simulink model "running_example"  (Simulink 10.0)
settings: Solver=ode45  StartTime=0.0  StopTime=50.0  RelTol=1e-3  EnableMultiTasking=on
settings Model: Creator=unknown  LastModifiedBy=bhisma
settings DataIOCC: LimitDataPoints=on  SignalLoggingSaveFormat=ModelDataLogs  SignalLoggingName=sigsOut
settings OptimizationCC: LifeSpan=auto
settings DebuggingCC: SaveWithParameterizedLinksMsg=none  SignalResolutionControl=TryResolveAllWithWarning  MultiTaskDSMMsg=warning  MultiTaskCondExecSysMsg=none  SFUnexpectedBacktrackingDiag=error  SFNoUnconditionalDefaultTransitionDiag=error  SFExecutionAtInitializationDiag=warning  ArithmeticOperatorsInVariantConditions=error
settings HardwareCC: TargetUnknown=on
settings SFSimCC: SimUseLocalCustomCode=on  CustomCodeUndefinedFunction=FilterOut
settings RTWCC: RTWUseLocalCustomCode=on
settings CodeAppCC: StateflowObjectComments=off
settings GRTTargetCC: TargetLangStandard=C99 (ISO)

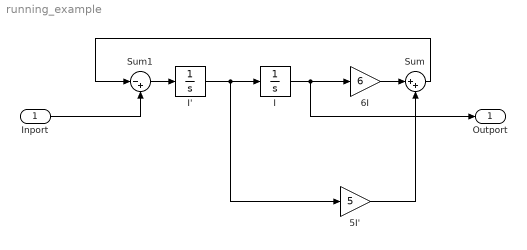
== system running_example ==
  Inport : Inport
  5I' : Gain  Gain=5  SaturateOnIntegerOverflow=on  OutDataTypeStr=Inherit: Same as input  ParamDataTypeStr=Inherit: Same as input
  6I : Gain  Gain=6  SaturateOnIntegerOverflow=on  OutDataTypeStr=Inherit: Same as input  ParamDataTypeStr=Inherit: Same as input
  I : Integrator  InitialCondition=1
  I' : Integrator  InitialCondition=5
  Sum : Sum  Inputs=|++  SaturateOnIntegerOverflow=on
  Sum1 : Sum  Inputs=|-+  SaturateOnIntegerOverflow=on
  Outport : Outport
  wires:
  I'/1 -> I/1, 5I'/1
  I/1 -> 6I/1, Outport/1
  6I/1 -> Sum/1
  Sum1/1 -> I'/1
  Inport/1 -> Sum1/2
  5I'/1 -> Sum/2
  Sum/1 -> Sum1/1
